simulink model "VoltageBias"  (R2018a)
settings: Solver=VariableStepAuto  StartTime=0.0  StopTime=10.0  RelTol=1e-3
values from neighbouring files (symbols this model uses):
  Ld = 450e-12    (= 4.5e-10)    [parameters.m]
  Lgin = 0.65e-9    (= 6.5e-10)    [parameters.m]
  Ls = 42e-12    (= 4.2e-11)    [parameters.m]
  Lss = 0.43e-9    (= 4.3e-10)    [parameters.m]
  Rd = (3.6/8) * (0.95*0.82*(1 - (-0.0135*(25 - 25))) * 18.2 / 295)    (= 0.0216271525424)    [parameters.m]
  Rgin = 1.5    [parameters.m]
  Rs = 3.6 * 0.238 * 0.82 * (1 - (-0.0135*(25 - 25))) / 295    (= 0.00238161355932)    [parameters.m]
  Rss = 1e-3    (= 0.001)    [parameters.m]
libraries: cstblocks x1
settings Model: Creator=enes_  LastModifiedBy=enes_

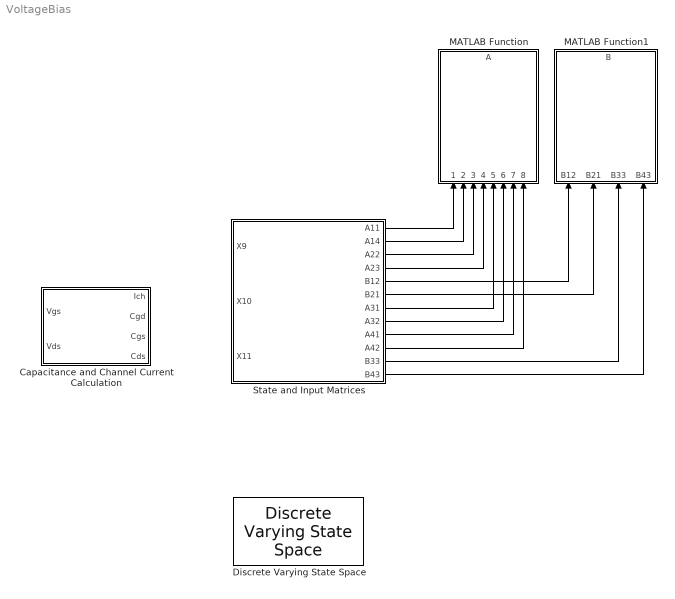
== system VoltageBias ==
  "Capacitance and Channel Current Calculation " : MATLAB Function  TreatAsAtomicUnit=on
  Discrete Varying State Space : cstblocks/Linear Parameter Varying/Discrete Varying State Space  x0=0  Ts=-1  OutputX=on  OutputDX=on
      settings: SourceProductName=Control System Toolbox  SourceProductBaseCode=CT
  MATLAB Function : MATLAB Function  TreatAsAtomicUnit=on
  MATLAB Function1 : MATLAB Function  TreatAsAtomicUnit=on
  State and Input Matrices : Subsystem
  wires:
  State and Input Matrices/1(A11) -> MATLAB Function/1(A11)
  State and Input Matrices/2(A14) -> MATLAB Function/2(A14)
  State and Input Matrices/3(A22) -> MATLAB Function/3(A22)
  State and Input Matrices/4(A23) -> MATLAB Function/4(A23)
  State and Input Matrices/7(A31) -> MATLAB Function/5(A31)
  State and Input Matrices/8(A32) -> MATLAB Function/6(A32)
  State and Input Matrices/9(A41) -> MATLAB Function/7(A41)
  State and Input Matrices/10(A42) -> MATLAB Function/8(A42)
  State and Input Matrices/5(B12) -> MATLAB Function1/1(B12)
  State and Input Matrices/6(B21) -> MATLAB Function1/2(B21)
  State and Input Matrices/11(B33) -> MATLAB Function1/3(B33)
  State and Input Matrices/12(B43) -> MATLAB Function1/4(B43)

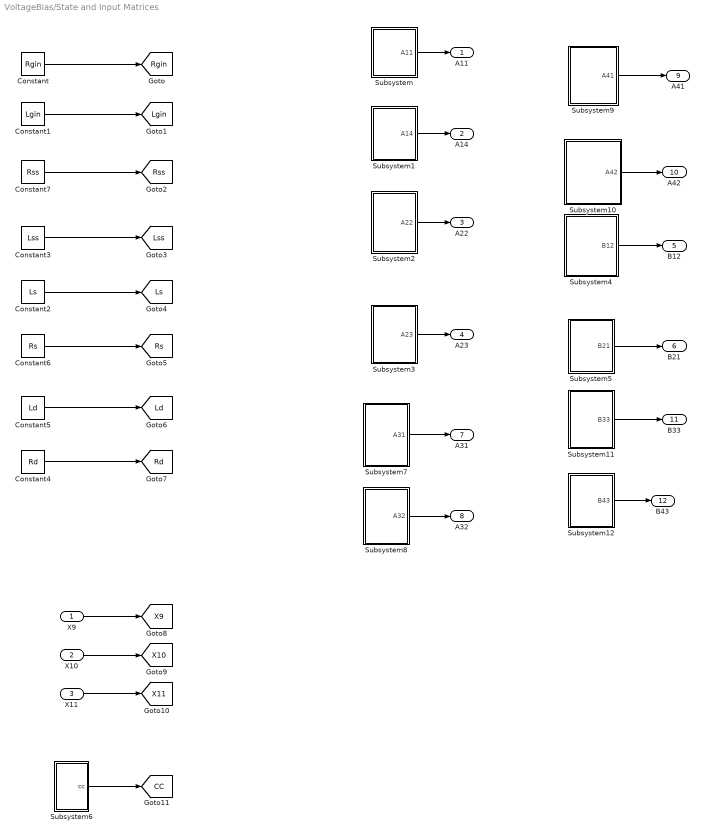
== system VoltageBias/State and Input Matrices ==
  X9 : Inport
  X10 : Inport  Port=2
  X11 : Inport  Port=3
  Constant : Constant  Value=Rgin
  Constant1 : Constant  Value=Lgin
  Constant2 : Constant  Value=Ls
  Constant3 : Constant  Value=Lss
  Constant4 : Constant  Value=Rd
  Constant5 : Constant  Value=Ld
  Constant6 : Constant  Value=Rs
  Constant7 : Constant  Value=Rss
  Subsystem : Subsystem
  Subsystem1 : Subsystem
  Subsystem10 : Subsystem
  Subsystem11 : Subsystem
  Subsystem12 : Subsystem
  Subsystem2 : Subsystem
  Subsystem3 : Subsystem
  Subsystem4 : Subsystem
  Subsystem5 : Subsystem
  Subsystem6 : Subsystem
  Subsystem7 : Subsystem
  Subsystem8 : Subsystem
  Subsystem9 : Subsystem
  A11 : Outport
  A14 : Outport  Port=2
  A22 : Outport  Port=3
  A23 : Outport  Port=4
  B12 : Outport  Port=5
  B21 : Outport  Port=6
  A31 : Outport  Port=7
  A32 : Outport  Port=8
  A41 : Outport  Port=9
  A42 : Outport  Port=10
  B33 : Outport  Port=11
  B43 : Outport  Port=12
  tag scope: CC=global, Ld=global, Lgin=global, Ls=global, Lss=global, Rd=global, Rgin=global, Rs=global, Rss=global, X10=global, X11=global, X9=global
  wires:
  Constant/1 -> [Rgin]
  Constant1/1 -> [Lgin]
  Constant7/1 -> [Rss]
  Constant3/1 -> [Lss]
  Constant2/1 -> [Ls]
  Constant6/1 -> [Rs]
  Constant5/1 -> [Ld]
  Constant4/1 -> [Rd]
  Subsystem/1(A11) -> A11/1
  Subsystem1/1(A14) -> A14/1
  Subsystem2/1(A22) -> A22/1
  Subsystem3/1(A23) -> A23/1
  Subsystem4/1(B12) -> B12/1
  Subsystem5/1(B21) -> B21/1
  X9/1 -> [X9]
  X10/1 -> [X10]
  X11/1 -> [X11]
  Subsystem6/1("cc ") -> [CC]
  Subsystem7/1(A31) -> A31/1
  Subsystem8/1(A32) -> A32/1
  Subsystem9/1(A41) -> A41/1
  Subsystem10/1(A42) -> A42/1
  Subsystem11/1(B33) -> B33/1
  Subsystem12/1(B43) -> B43/1

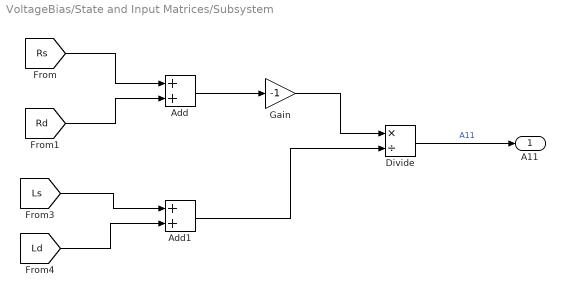
== system VoltageBias/State and Input Matrices/Subsystem ==
  Add : Sum
  Add1 : Sum
  Divide : Product  Inputs=*/
  Gain : Gain  Gain=-1
  A11 : Outport
  wires:
  Add1/1 -> Divide/2
  [Rd] -> Add/2
  [Ls] -> Add1/1
  Divide/1 -> A11/1  "A11"
  [Rs] -> Add/1
  Add/1 -> Gain/1
  [Ld] -> Add1/2
  Gain/1 -> Divide/1

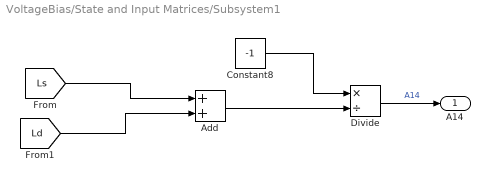
== system VoltageBias/State and Input Matrices/Subsystem1 ==
  Add : Sum
  Constant8 : Constant  Value=-1
  Divide : Product  Inputs=*/
  A14 : Outport
  wires:
  Divide/1 -> A14/1  "A14"
  Add/1 -> Divide/2
  Constant8/1 -> Divide/1
  [Ld] -> Add/2
  [Ls] -> Add/1

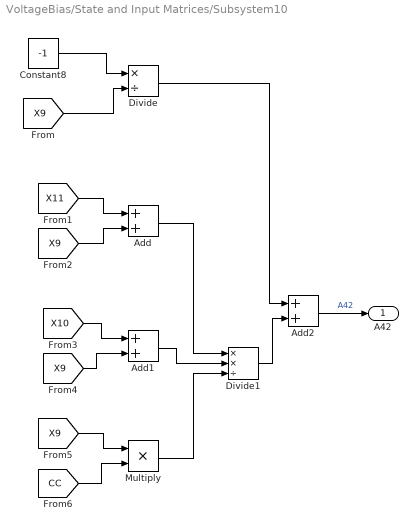
== system VoltageBias/State and Input Matrices/Subsystem10 ==
  Add : Sum
  Add1 : Sum
  Add2 : Sum
  Constant8 : Constant  Value=-1
  Divide : Product  Inputs=*/
  Divide1 : Product  Inputs=**/
  Multiply : Product
  A42 : Outport
  wires:
  Divide1/1 -> Add2/2
  [X11] -> Add/1
  Add1/1 -> Divide1/2
  [X10] -> Add1/1
  Constant8/1 -> Divide/1
  [CC] -> Multiply/2
  [X9] -> Add/2
  [X9] -> Add1/2
  [X9] -> Multiply/1
  [X9] -> Divide/2
  Multiply/1 -> Divide1/3
  Divide/1 -> Add2/1
  Add/1 -> Divide1/1
  Add2/1 -> A42/1  "A42"

== system VoltageBias/State and Input Matrices/Subsystem11 ==
  Constant8 : Constant  Value=-1
  Divide : Product  Inputs=**/
  B33 : Outport
  wires:
  Divide/1 -> B33/1  "B33"
  [CC] -> Divide/3
  [X9] -> Divide/2
  Constant8/1 -> Divide/1

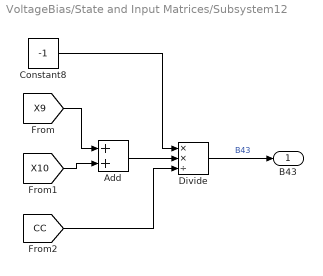
== system VoltageBias/State and Input Matrices/Subsystem12 ==
  Add : Sum
  Constant8 : Constant  Value=-1
  Divide : Product  Inputs=**/
  B43 : Outport
  wires:
  [CC] -> Divide/3
  [X10] -> Add/2
  Add/1 -> Divide/2
  Divide/1 -> B43/1  "B43"
  [X9] -> Add/1
  Constant8/1 -> Divide/1

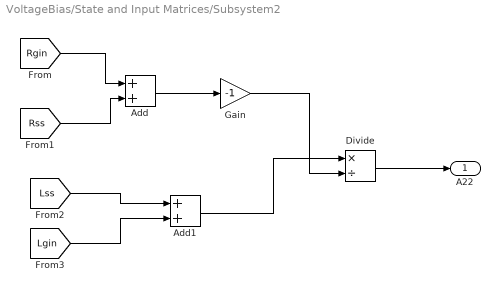
== system VoltageBias/State and Input Matrices/Subsystem2 ==
  Add : Sum
  Add1 : Sum
  Divide : Product  Inputs=*/
  Gain : Gain  Gain=-1
  A22 : Outport
  wires:
  Gain/1 -> Divide/2
  Divide/1 -> A22/1
  [Rss] -> Add/2
  [Lss] -> Add1/1
  [Lgin] -> Add1/2
  [Rgin] -> Add/1
  Add1/1 -> Divide/1
  Add/1 -> Gain/1

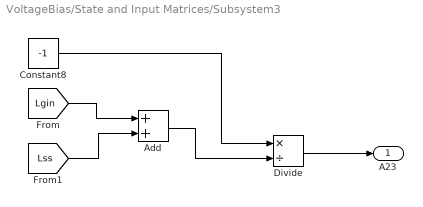
== system VoltageBias/State and Input Matrices/Subsystem3 ==
  Add : Sum
  Constant8 : Constant  Value=-1
  Divide : Product  Inputs=*/
  A23 : Outport
  wires:
  Add/1 -> Divide/2
  Constant8/1 -> Divide/1
  [Lgin] -> Add/1
  [Lss] -> Add/2
  Divide/1 -> A23/1

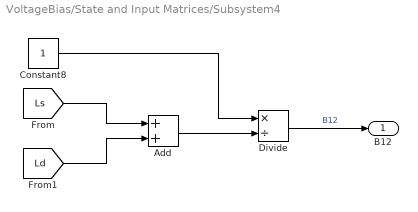
== system VoltageBias/State and Input Matrices/Subsystem4 ==
  Add : Sum
  Constant8 : Constant
  Divide : Product  Inputs=*/
  B12 : Outport
  wires:
  [Ls] -> Add/1
  Add/1 -> Divide/2
  [Ld] -> Add/2
  Constant8/1 -> Divide/1
  Divide/1 -> B12/1  "B12"

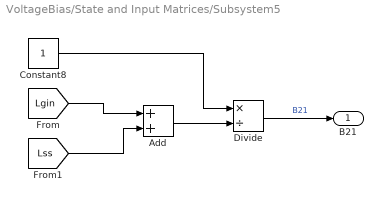
== system VoltageBias/State and Input Matrices/Subsystem5 ==
  Add : Sum
  Constant8 : Constant
  Divide : Product  Inputs=*/
  B21 : Outport
  wires:
  Constant8/1 -> Divide/1
  Divide/1 -> B21/1  "B21"
  [Lgin] -> Add/1
  Add/1 -> Divide/2
  [Lss] -> Add/2

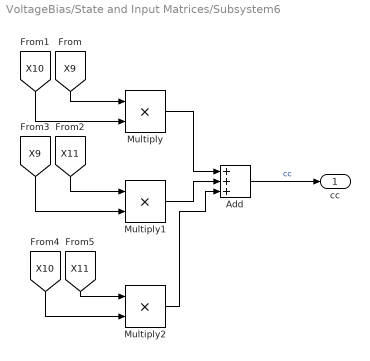
== system VoltageBias/State and Input Matrices/Subsystem6 ==
  Add : Sum  Inputs=3
  Multiply : Product
  Multiply1 : Product
  Multiply2 : Product
  "cc " : Outport
  wires:
  Multiply/1 -> Add/1
  [X9] -> Multiply/1
  [X9] -> Multiply1/2
  [X10] -> Multiply/2
  Multiply2/1 -> Add/3
  Add/1 -> "cc "/1  "cc"
  [X11] -> Multiply1/1
  [X10] -> Multiply2/2
  Multiply1/1 -> Add/2
  [X11] -> Multiply2/1

== system VoltageBias/State and Input Matrices/Subsystem7 ==
  Divide : Product  Inputs=*/
  A31 : Outport
  wires:
  [X9] -> Divide/1
  [CC] -> Divide/2
  Divide/1 -> A31/1  "A31"

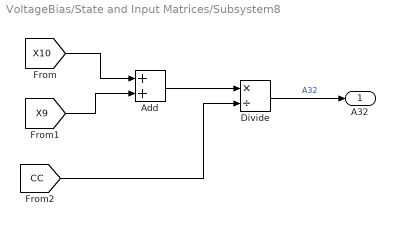
== system VoltageBias/State and Input Matrices/Subsystem8 ==
  Add : Sum
  Divide : Product  Inputs=*/
  A32 : Outport
  wires:
  Add/1 -> Divide/1
  Divide/1 -> A32/1  "A32"
  [X10] -> Add/1
  [X9] -> Add/2
  [CC] -> Divide/2

== system VoltageBias/State and Input Matrices/Subsystem9 ==
  Add : Sum
  Divide : Product  Inputs=*/
  A41 : Outport
  wires:
  [X10] -> Add/2
  Add/1 -> Divide/1
  Divide/1 -> A41/1  "A41"
  [X9] -> Add/1
  [CC] -> Divide/2

== matlab function VoltageBias/MATLAB Function ==
  data: A11 input; A output; A14 input; A22 input; A23 input; A31 input; A32 input; A41 input; A42 input
function A = StateMatrix(A11,A14,A22,A23,A31,A32,A41,A42)

x=zeros(4);

x(1,1)= A11;
x(1,4)= A14;
x(2,2)= A22;
x(2,3)= A23;
x(3,1)= A31;
x(3,2)= A32;
x(4,1)= A41;
x(4,2)= A42;

A=x;

== matlab function VoltageBias/Capacitance and Channel Current Calculation  ==
  data: Vgs input; Ich output; Vds input; Cgd output; Cgs output; Cds output
function [Ich,Cgd,Cgs,Cds] = NumericCalc(Vgs,Vds) %Vgin,Vdin,Vsin
% Vgs = x5-x4;
% Vds = x4-x3;
% Vgd = x5-x4;
Vgd = Vgs - Vds;
cur = 4.5057; % To be updated
K = cur * 0.8 * (273/300)^(-2.7);
x0 = 0.31 ;
x1 = 0.255;
slp = 2;
if Vds>=0
            Ich = K*log(1+exp(26*(Vgs-1.7)/slp))*(Vds)/(1+max((x0+x1*(Vgs+4.1)),0.2)*Vds);
else
            Ich = -K*log(1+exp(26*(Vgd-1.7)/slp))*(-Vds)/(1+max((x0+x1*(Vgd+6.1)),0.2)*(-Vds));
end

Vds = abs(Vds);
%% Crss Calc
 if Vds<=51
     Crss = -1.0716*Vds + 56.3216;
 else
     Crss = 1.67;
 end
 Crss = Crss * 1e-12;
%% Coss Calc
if Vds <= 40
    Coss = -1.60513*Vds+500.11;
elseif Vds<=70
    Coss = -8.563*Vds+778.41; 
elseif Vds<=222
    Coss = -0.6711*Vds+226;
else
    Coss = -0.0534*Vds+88.86;
end
 Coss = Coss * 1e-12;
%% Ciss Calc

if Vgs <= 1
    Ciss = 9.245*Vds+231.35;
elseif Vgs<=2
    Ciss = 400.9*Vgs+641.5; 
elseif Vgs<=5
    Ciss = -37*Vgs+715.5;
else
    Ciss = -9.4*Vgs+577.5;
end
 Ciss = Ciss * 1e-12;

%% Outputs
Cgs = Ciss - Crss;
Cds = Coss - Crss;
Cgd = Crss;
% 
% end

== matlab function VoltageBias/MATLAB Function1 ==
  data: B12 input; B output; B21 input; B33 input; B43 input
function B = InputMatrix(B12, B21,B33,B43)
x=zeros(4);

x(1,2)= B12;
x(2,1)= B21;
x(3,3)= B33;
x(4,3)= B43;

B=x;
